simulink model "Robust_joint_Space"  (R2020b)
settings: Solver=VariableStepAuto  StartTime=0.0  StopTime=10  RelTol=1e-3
(part 4 of 7)

== matlab function Robust_joint_Space/plant/MATLAB Function4 ==
  data: M input; NumTerm input; Thetadd output
function Thetadd = Response(M,NumTerm)
Thetadd=M\NumTerm;

== matlab function Robust_joint_Space/plant/MATLAB Function2 ==
  data: Theta input; M output
function M = NumM(Theta)
t1=Theta(1);
t2=Theta(2);
t3=Theta(3);
t4=Theta(4);
t5=Theta(5);
t6=Theta(6);

L1=0.1025;
L2=0.408;
L3=0.376;
L4=0.1025; 
L5=0.1025;


M=zeros(6);
M(1)=(999498*cos(t3 + t4))/5 - (9799*L4)/40 - (33481296*cos(2*t2 + t3))/25 -...
    (30203396714246934648101547*cos(2*t2))/28823037615171174400 - (401759*cos(2*t2 + 2*t3 + 2*t4))/16 -...
    (15427656*cos(2*t2 + 2*t3))/25 - (999498*cos(2*t2 + t3 + t4))/5 - (219461*L1)/100 + (33481296*cos(t3))/25 +...
    (921106*cos(t4))/5 - (921106*cos(2*t2 + 2*t3 + t4))/5 - (239*L3^2*cos(2*t2 + 2*t3 + 2*t4 - 2*t5))/3200 -...
    (239*L3^2*cos(2*t2 + 2*t3 + 2*t4 + 2*t5))/3200 + (24378*L4*cos(2*t2 + t3 + t4))/25 +...
    (12189*L3*cos(t3 + t4 - t5))/50 - (757*L2^2*cos(2*t2))/800 + (239*L3^2*cos(2*t5))/1600 +...
    (239*L3^2*cos(2*t2 + 2*t3 + 2*t4))/1600 - (239*L4^2*cos(2*t2 + 2*t3 + 2*t4))/200 - (24378*L4*cos(t3 + t4))/25 -...
    (11233*L3*cos(t4 + t5))/50 - (11233*L3*cos(2*t2 + 2*t3 + t4 - t5))/50 + (9799*L3*cos(2*t2 + 2*t3 + 2*t4 + t5))/160 +...
    (67159*L3*cos(t5))/200 - (22466*L4*cos(t4))/25 + (22466*L4*cos(2*t2 + 2*t3 + t4))/25 +...
    (12189*L3*cos(2*t2 + t3 + t4 + t5))/50 + (781*L1^2)/100 + (757*L2^2)/800 + (717*L3^2)/1600 +...
    (239*L4^2)/200 + (11233*L3*cos(t4 - t5))/50 - (9799*L3*cos(2*t2 + 2*t3 + 2*t4 - t5))/160 -...
    (12189*L3*cos(t3 + t4 + t5))/50 + (9799*L4*cos(2*t2 + 2*t3 + 2*t4))/40 -...
    (12189*L3*cos(2*t2 + t3 + t4 - t5))/50 + (11233*L3*cos(2*t2 + 2*t3 + t4 + t5))/50 +...
    (239*L3*L4*cos(2*t2 + 2*t3 + 2*t4 - t5))/400 - (239*L3*L4*cos(2*t2 + 2*t3 + 2*t4 + t5))/400 +...
    60184539611691967063155889/28823037615171174400;
M(7)=(61463515545781917*cos(t1 + 2*t2))/2305843009213693952 - (61463515545781917*cos(t1 - 2*t2))/2305843009213693952 -...
    (2753519*cos(t2 + t3 + t4))/40 - (11529711*cos(t2 + t3))/25 - (18042729*cos(t2))/25 - (757*L2^2*cos(t1 - 2*t2))/1600 +...
    (757*L2^2*cos(t1 + 2*t2))/1600 - (11233*L3*cos(t2 + t3 - t5))/50 + (4541*L3*cos(t2 + t3 + t4 + t5))/200 -...
    (212717*L2*cos(t1 + t2))/800 + (7426*L1*cos(t2 + t3))/5 - (12189*L3*cos(t2 + t5))/50 + (79662*L1*cos(t2))/25 -...
    (58077*L3*cos(t2 + t3 + t4 - t5))/400 - (212717*L2*cos(t1 - t2))/800 - (12189*L3*cos(t2 - t5))/50 -...
    (11233*L3*cos(t2 + t3 + t5))/50 + (67159*L4*cos(t2 + t3 + t4))/200 - (239*L3^2*cos(t2 + t3 + t4 - 2*t5))/1600 +...
    (239*L3^2*cos(t2 + t3 + t4 + 2*t5))/1600 + (239*L3*L4*cos(t2 + t3 + t4 + t5))/400 +...
    (239*L3*L4*cos(t2 + t3 + t4 - t5))/400;
M(13)=(1690603261718859*cos(t1 - 2*t2))/2305843009213693952 - (1690603261718859*cos(t1 + 2*t2))/2305843009213693952 -...
    (2753519*cos(t2 + t3 + t4))/40 - (11529711*cos(t2 + t3))/25 - (11233*L3*cos(t2 + t3 - t5))/50 +...
    (4541*L3*cos(t2 + t3 + t4 + t5))/200 + (7426*L1*cos(t2 + t3))/5 - (58077*L3*cos(t2 + t3 + t4 - t5))/400 -...
    (11233*L3*cos(t2 + t3 + t5))/50 + (67159*L4*cos(t2 + t3 + t4))/200 - (239*L3^2*cos(t2 + t3 + t4 - 2*t5))/1600 +...
    (239*L3^2*cos(t2 + t3 + t4 + 2*t5))/1600 + (239*L3*L4*cos(t2 + t3 + t4 + t5))/400 +...
    (239*L3*L4*cos(t2 + t3 + t4 - t5))/400;
M(19)=(1690603261718859*cos(t1 - 2*t2))/2305843009213693952 - (1690603261718859*cos(t1 + 2*t2))/2305843009213693952 -...
    (2753519*cos(t2 + t3 + t4))/40 + (4541*L3*cos(t2 + t3 + t4 + t5))/200 - (58077*L3*cos(t2 + t3 + t4 - t5))/400 +...
    (67159*L4*cos(t2 + t3 + t4))/200 - (239*L3^2*cos(t2 + t3 + t4 - 2*t5))/1600 + (239*L3^2*cos(t2 + t3 + t4 + 2*t5))/1600 +...
    (239*L3*L4*cos(t2 + t3 + t4 + t5))/400 + (239*L3*L4*cos(t2 + t3 + t4 - t5))/400;
M(25)=(1690603261718859*cos(t2 + t3 + t4))/1152921504606846976 - (1690603261718859*cos(t1 + t2 - t3 - t4))/4611686018427387904 +...
    (1690603261718859*cos(3*t2 - t1 + t3 + t4))/4611686018427387904 - (1690603261718859*cos(t3 - t2 + t4))/2305843009213693952 -...
    (1690603261718859*cos(3*t2 + t3 + t4))/2305843009213693952 - (1690603261718859*cos(t1 - t2 + t3 + t4))/4611686018427387904 +...
    (1690603261718859*cos(t1 + 3*t2 + t3 + t4))/4611686018427387904 - (11233*L3*cos(t2 + t3 - t5))/50 + (239*L3^2*cos(t2 + t3 + t4))/400 +...
    (58077*L3*cos(t2 + t3 + t4 + t5))/400 + (12189*L3*cos(t2 + t5))/50 + (4541*L3*cos(t2 + t3 + t4 - t5))/200 - (12189*L3*cos(t2 - t5))/50 +...
    (11233*L3*cos(t2 + t3 + t5))/50 - (239*L3*L4*cos(t2 + t3 + t4 + t5))/400 + (239*L3*L4*cos(t2 + t3 + t4 - t5))/400;
M(31)=0;
M(2)=(61463515545781917*cos(t1 + 2*t2))/2305843009213693952 - (61463515545781917*cos(t1 - 2*t2))/2305843009213693952 -...
    (2753519*cos(t2 + t3 + t4))/40 - (11529711*cos(t2 + t3))/25 - (18042729*cos(t2))/25 - (757*L2^2*cos(t1 - 2*t2))/1600 +...
    (757*L2^2*cos(t1 + 2*t2))/1600 - (11233*L3*cos(t2 + t3 - t5))/50 + (4541*L3*cos(t2 + t3 + t4 + t5))/200 -...
    (212717*L2*cos(t1 + t2))/800 + (7426*L1*cos(t2 + t3))/5 - (12189*L3*cos(t2 + t5))/50 + (79662*L1*cos(t2))/25 -...
    (58077*L3*cos(t2 + t3 + t4 - t5))/400 - (212717*L2*cos(t1 - t2))/800 - (12189*L3*cos(t2 - t5))/50 -...
    (11233*L3*cos(t2 + t3 + t5))/50 + (67159*L4*cos(t2 + t3 + t4))/200 - (239*L3^2*cos(t2 + t3 + t4 - 2*t5))/1600 +...
    (239*L3^2*cos(t2 + t3 + t4 + 2*t5))/1600 + (239*L3*L4*cos(t2 + t3 + t4 + t5))/400 + (239*L3*L4*cos(t2 + t3 + t4 - t5))/400;
M(8)=(66962592*cos(t3))/25 - (9799*L4)/20 + (1842212*cos(t4))/5 + (1998996*cos(t3)*cos(t4))/5 - (1998996*sin(t3)*sin(t4))/5 -...
    (17228543827841635967893663*cos(t1)^2)/115292150460684697600 - (61463515545781917*cos(t2)^2)/576460752303423488 +...
    (1690603261718859*cos(t3)^2)/576460752303423488 + (757*L2^2*cos(t1)^2)/400 + (757*L2^2*cos(t2)^2)/400 -...
    (239*L3^2*cos(t5)^2)/400 - (44932*L4*cos(t4))/25 + (239*L3^2)/400 + (239*L4^2)/100 + ...
    (61463515545781917*cos(t1)^2*cos(t2)^2)/576460752303423488 - (1690603261718859*cos(t1)^2*cos(t3)^2)/288230376151711744 -...
    (48756*L4*cos(t3)*cos(t4))/25 - (757*L2^2*cos(t1)^2*cos(t2)^2)/400 + (48756*L4*sin(t3)*sin(t4))/25 + (22466*L3*sin(t4)*sin(t5))/25 -...
    (212717*L2*cos(t1)*sin(t1)*sin(t2))/200 + (24378*L3*cos(t3)*sin(t4)*sin(t5))/25 + (24378*L3*cos(t4)*sin(t3)*sin(t5))/25 -...
    (1690603261718859*cos(t1)*cos(t3)*sin(t1)*sin(t3))/288230376151711744 + 406940712223380376880235337/115292150460684697600;
M(14)=(33481296*cos(t3))/25 - (9799*L4)/20 + (1842212*cos(t4))/5 + (999498*cos(t3)*cos(t4))/5 - (999498*sin(t3)*sin(t4))/5 +...
    (22503512638915017*cos(t1)^2)/4611686018427387904 + (1690603261718859*cos(t2)^2)/576460752303423488 +...
    (1690603261718859*cos(t3)^2)/576460752303423488 - (239*L3^2*cos(t5)^2)/400 - (44932*L4*cos(t4))/25 +...
    (239*L3^2)/400 + (239*L4^2)/100 - (1690603261718859*cos(t1)^2*cos(t2)^2)/576460752303423488 -...
    (1690603261718859*cos(t1)^2*cos(t3)^2)/288230376151711744 - (24378*L4*cos(t3)*cos(t4))/25 +...
    (24378*L4*sin(t3)*sin(t4))/25 + (22466*L3*sin(t4)*sin(t5))/25 + (12189*L3*cos(t3)*sin(t4)*sin(t5))/25 +...
    (12189*L3*cos(t4)*sin(t3)*sin(t5))/25 - (1690603261718859*cos(t1)*cos(t3)*sin(t1)*sin(t3))/288230376151711744 +...
    148084969195448577098115273/115292150460684697600;
M(20)=(24162136260015883*cos(2*t1))/9223372036854775808 - (9799*L4)/20 + (1690603261718859*cos(2*t2))/2305843009213693952 +...
    (921106*cos(t4))/5 + (999498*cos(t3)*cos(t4))/5 - (999498*sin(t3)*sin(t4))/5 - (239*L3^2*cos(t5)^2)/400 -...
    (22466*L4*cos(t4))/25 + (239*L3^2)/400 + (239*L4^2)/100 - (1690603261718859*cos(2*t1)*cos(2*t2))/2305843009213693952 -...
    (1690603261718859*cos(2*t1)*cos(t3)^2)/576460752303423488 - (24378*L4*cos(t3)*cos(t4))/25 -...
    (1690603261718859*sin(2*t1)*cos(t3)*sin(t3))/576460752303423488 + (24378*L4*sin(t3)*sin(t4))/25 +...
    (11233*L3*sin(t4)*sin(t5))/25 + (12189*L3*cos(t3)*sin(t4)*sin(t5))/25 + (12189*L3*cos(t4)*sin(t3)*sin(t5))/25 +...
    463196680911590935827689/9223372036854775808;
M(26)=(1690603261718859*cos(2*t1 + t2 - t3 + t4))/2305843009213693952 - (1690603261718859*cos(t1 + t2 - t3 - t4))/4611686018427387904 +...
    (1690603261718859*cos(2*t1 - t2 + t3 + t4))/9223372036854775808 + (1690603261718859*cos(3*t2 - t1 + t3 + t4))/4611686018427387904 -...
    (1690603261718859*cos(t2 - 2*t1 + 3*t3 + t4))/2305843009213693952 - (1690603261718859*cos(3*t2 - 2*t1 + t3 + t4))/9223372036854775808 +...
    (1690603261718859*cos(2*t1 + 3*t2 + t3 + t4))/9223372036854775808 - (1690603261718859*cos(2*t1 + t2 - t3 - t4))/9223372036854775808 +...
    (1690603261718859*cos(t1 - t2 + t3 + t4))/4611686018427387904 + (10637310166265011*cos(t2 - 2*t1 + t3 + t4))/18446744073709551616 -...
    (10637310166265011*cos(2*t1 + t2 + t3 + t4))/18446744073709551616 - (1690603261718859*cos(t1 + 3*t2 + t3 + t4))/4611686018427387904 -...
    (12189*L3*cos(t3 + t4 - t5))/50 - (11233*L3*cos(t4 + t5))/50 - (9799*L3*cos(t5))/80 - (11233*L3*cos(t4 - t5))/50 -...
    (12189*L3*cos(t3 + t4 + t5))/50 + (239*L3*L4*cos(t5))/200;
M(32)=(3874897119389575*cos(t5))/4611686018427387904 + (3874897119389575*cos(t1)^2*cos(t5))/4611686018427387904 -...
    (3874897119389575*cos(t1)*cos(t2)*cos(t3)*cos(t4)*sin(t1)*sin(t5))/4611686018427387904 +...
    (3874897119389575*cos(t1)*cos(t2)*sin(t1)*sin(t3)*sin(t4)*sin(t5))/4611686018427387904 +...
    (3874897119389575*cos(t1)*cos(t3)*sin(t1)*sin(t2)*sin(t4)*sin(t5))/4611686018427387904 +...
    (3874897119389575*cos(t1)*cos(t4)*sin(t1)*sin(t2)*sin(t3)*sin(t5))/4611686018427387904;
M(3)=(1690603261718859*cos(t1 - 2*t2))/2305843009213693952 - (1690603261718859*cos(t1 + 2*t2))/2305843009213693952 -...
    (2753519*cos(t2 + t3 + t4))/40 - (11529711*cos(t2 + t3))/25 - (11233*L3*cos(t2 + t3 - t5))/50 +...
    (4541*L3*cos(t2 + t3 + t4 + t5))/200 + (7426*L1*cos(t2 + t3))/5 - (58077*L3*cos(t2 + t3 + t4 - t5))/400 -...
    (11233*L3*cos(t2 + t3 + t5))/50 + (67159*L4*cos(t2 + t3 + t4))/200 - (239*L3^2*cos(t2 + t3 + t4 - 2*t5))/1600 +...
    (239*L3^2*cos(t2 + t3 + t4 + 2*t5))/1600 + (239*L3*L4*cos(t2 + t3 + t4 + t5))/400 +...
    (239*L3*L4*cos(t2 + t3 + t4 - t5))/400;
M(9)=(33481296*cos(t3))/25 - (9799*L4)/20 + (1842212*cos(t4))/5 + (999498*cos(t3)*cos(t4))/5 - (999498*sin(t3)*sin(t4))/5 +...
    (22503512638915017*cos(t1)^2)/4611686018427387904 + (1690603261718859*cos(t2)^2)/576460752303423488 + ...
    (1690603261718859*cos(t3)^2)/576460752303423488 - (239*L3^2*cos(t5)^2)/400 - (44932*L4*cos(t4))/25 + ...
    (239*L3^2)/400 + (239*L4^2)/100 - (1690603261718859*cos(t1)^2*cos(t2)^2)/576460752303423488 - ...
    (1690603261718859*cos(t1)^2*cos(t3)^2)/288230376151711744 - (24378*L4*cos(t3)*cos(t4))/25 + ...
    (24378*L4*sin(t3)*sin(t4))/25 + (22466*L3*sin(t4)*sin(t5))/25 + (12189*L3*cos(t3)*sin(t4)*sin(t5))/25 +...
    (12189*L3*cos(t4)*sin(t3)*sin(t5))/25 - (1690603261718859*cos(t1)*cos(t3)*sin(t1)*sin(t3))/288230376151711744 +...
    148084969195448577098115273/115292150460684697600;
M(15)=(1842212*cos(t4))/5 - (9799*L4)/20 + (22503512638915017*cos(t1)^2)/4611686018427387904 +...
    (1690603261718859*cos(t2)^2)/576460752303423488 + (1690603261718859*cos(t3)^2)/576460752303423488 -...
    (239*L3^2*cos(t5)^2)/400 - (44932*L4*cos(t4))/25 + (239*L3^2)/400 + (239*L4^2)/100 -...
    (1690603261718859*cos(t1)^2*cos(t2)^2)/576460752303423488 - (1690603261718859*cos(t1)^2*cos(t3)^2)/288230376151711744 +...
    (22466*L3*sin(t4)*sin(t5))/25 - (1690603261718859*cos(t1)*cos(t3)*sin(t1)*sin(t3))/288230376151711744 +...
    148084969195448577098115273/115292150460684697600;
M(21)=(921106*cos(t4))/5 - (9799*L4)/20 + (30924549306891319*cos(t1)^2)/4611686018427387904 +...
    (1690603261718859*cos(t2)^2)/576460752303423488 + (1690603261718859*cos(t3)^2)/576460752303423488 -...
    (239*L3^2*cos(t5)^2)/400 - (22466*L4*cos(t4))/25 + (239*L3^2)/400 + (239*L4^2)/100 -...
    (1690603261718859*cos(t1)^2*cos(t2)^2)/576460752303423488 - (1690603261718859*cos(t1)^2*cos(t3)^2)/288230376151711744 +...
    (11233*L3*sin(t4)*sin(t5))/25 - (1690603261718859*cos(t1)*cos(t3)*sin(t1)*sin(t3))/288230376151711744 + 231598321612314291030467/4611686018427387904;
M(27)=(1690603261718859*cos(2*t1 + t2 - t3 + t4))/2305843009213693952 - (1690603261718859*cos(t1 + t2 - t3 - t4))/4611686018427387904 +...
    (1690603261718859*cos(2*t1 - t2 + t3 + t4))/9223372036854775808 + (1690603261718859*cos(3*t2 - t1 + t3 + t4))/4611686018427387904 -...
    (1690603261718859*cos(t2 - 2*t1 + 3*t3 + t4))/2305843009213693952 - (1690603261718859*cos(3*t2 - 2*t1 + t3 + t4))/9223372036854775808 +...
    (1690603261718859*cos(2*t1 + 3*t2 + t3 + t4))/9223372036854775808 - (1690603261718859*cos(2*t1 + t2 - t3 - t4))/9223372036854775808 +...
    (1690603261718859*cos(t1 - t2 + t3 + t4))/4611686018427387904 + (10637310166265011*cos(t2 - 2*t1 + t3 + t4))/18446744073709551616 -...
    (10637310166265011*cos(2*t1 + t2 + t3 + t4))/18446744073709551616 - (1690603261718859*cos(t1 + 3*t2 + t3 + t4))/4611686018427387904 -...
    (11233*L3*cos(t4 + t5))/50 - (9799*L3*cos(t5))/80 - (11233*L3*cos(t4 - t5))/50 + (239*L3*L4*cos(t5))/200;
M(33)=(3874897119389575*cos(t5))/4611686018427387904 + (3874897119389575*cos(t1)^2*cos(t5))/4611686018427387904 -...
    (3874897119389575*cos(t1)*cos(t2)*cos(t3)*cos(t4)*sin(t1)*sin(t5))/4611686018427387904 +...
    (3874897119389575*cos(t1)*cos(t2)*sin(t1)*sin(t3)*sin(t4)*sin(t5))/4611686018427387904 +...
    (3874897119389575*cos(t1)*cos(t3)*sin(t1)*sin(t2)*sin(t4)*sin(t5))/4611686018427387904 +...
    (3874897119389575*cos(t1)*cos(t4)*sin(t1)*sin(t2)*sin(t3)*sin(t5))/4611686018427387904;
M(4)=(1690603261718859*cos(t1 - 2*t2))/2305843009213693952 - (1690603261718859*cos(t1 + 2*t2))/2305843009213693952 -...
    (2753519*cos(t2 + t3 + t4))/40 + (4541*L3*cos(t2 + t3 + t4 + t5))/200 - (58077*L3*cos(t2 + t3 + t4 - t5))/400 +...
    (67159*L4*cos(t2 + t3 + t4))/200 - (239*L3^2*cos(t2 + t3 + t4 - 2*t5))/1600 + (239*L3^2*cos(t2 + t3 + t4 + 2*t5))/1600 +...
    (239*L3*L4*cos(t2 + t3 + t4 + t5))/400 + (239*L3*L4*cos(t2 + t3 + t4 - t5))/400;
M(10)=(24162136260015883*cos(2*t1))/9223372036854775808 - (9799*L4)/20 + (1690603261718859*cos(2*t2))/2305843009213693952 +...
    (921106*cos(t4))/5 + (999498*cos(t3)*cos(t4))/5 - (999498*sin(t3)*sin(t4))/5 - (239*L3^2*cos(t5)^2)/400 - (22466*L4*cos(t4))/25 +...
    (239*L3^2)/400 + (239*L4^2)/100 - (1690603261718859*cos(2*t1)*cos(2*t2))/2305843009213693952 -...
    (1690603261718859*cos(2*t1)*cos(t3)^2)/576460752303423488 - (24378*L4*cos(t3)*cos(t4))/25 -...
    (1690603261718859*sin(2*t1)*cos(t3)*sin(t3))/576460752303423488 + (24378*L4*sin(t3)*sin(t4))/25 + (11233*L3*sin(t4)*sin(t5))/25 +...
    (12189*L3*cos(t3)*sin(t4)*sin(t5))/25 + (12189*L3*cos(t4)*sin(t3)*sin(t5))/25 + 463196680911590935827689/9223372036854775808;
M(16)=(921106*cos(t4))/5 - (9799*L4)/20 + (30924549306891319*cos(t1)^2)/4611686018427387904 +...
    (1690603261718859*cos(t2)^2)/576460752303423488 + (1690603261718859*cos(t3)^2)/576460752303423488 -...
    (239*L3^2*cos(t5)^2)/400 - (22466*L4*cos(t4))/25 + (239*L3^2)/400 + (239*L4^2)/100 -...
    (1690603261718859*cos(t1)^2*cos(t2)^2)/576460752303423488 - (1690603261718859*cos(t1)^2*cos(t3)^2)/288230376151711744 +...
    (11233*L3*sin(t4)*sin(t5))/25 - (1690603261718859*cos(t1)*cos(t3)*sin(t1)*sin(t3))/288230376151711744 +...
    231598321612314291030467/4611686018427387904;
M(22)=(10637310166265011*cos(2*t1))/9223372036854775808 - (9799*L4)/20 + (1690603261718859*cos(2*t2))/2305843009213693952 -...
    (239*L3^2*cos(2*t5))/800 + (239*L3^2)/800 + (239*L4^2)/100 - (1690603261718859*cos(2*t1)*cos(2*t2))/2305843009213693952 -...
    (1690603261718859*cos(2*t1)*cos(2*t3))/1152921504606846976 - (1690603261718859*sin(2*t1)*sin(2*t3))/1152921504606846976 +...
    463196680911590935827689/9223372036854775808;
M(28)=(1690603261718859*cos(2*t1 + t2 - t3 + t4))/2305843009213693952 - (1690603261718859*cos(t1 + t2 - t3 - t4))/4611686018427387904 +...
    (1690603261718859*cos(2*t1 - t2 + t3 + t4))/9223372036854775808 + (1690603261718859*cos(3*t2 - t1 + t3 + t4))/4611686018427387904 -...
    (1690603261718859*cos(t2 - 2*t1 + 3*t3 + t4))/2305843009213693952 - (1690603261718859*cos(3*t2 - 2*t1 + t3 + t4))/9223372036854775808 +...
    (1690603261718859*cos(2*t1 + 3*t2 + t3 + t4))/9223372036854775808 - (1690603261718859*cos(2*t1 + t2 - t3 - t4))/9223372036854775808 +...
    (1690603261718859*cos(t1 - t2 + t3 + t4))/4611686018427387904 + (10637310166265011*cos(t2 - 2*t1 + t3 + t4))/18446744073709551616 -...
    (10637310166265011*cos(2*t1 + t2 + t3 + t4))/18446744073709551616 - (1690603261718859*cos(t1 + 3*t2 + t3 + t4))/4611686018427387904 -...
    (9799*L3*cos(t5))/80 + (239*L3*L4*cos(t5))/200;
M(34)=(3874897119389575*cos(t5))/4611686018427387904 + (3874897119389575*cos(t1)^2*cos(t5))/4611686018427387904 -...
    (3874897119389575*cos(t1)*cos(t2)*cos(t3)*cos(t4)*sin(t1)*sin(t5))/4611686018427387904 +...
    (3874897119389575*cos(t1)*cos(t2)*sin(t1)*sin(t3)*sin(t4)*sin(t5))/4611686018427387904 +...
    (3874897119389575*cos(t1)*cos(t3)*sin(t1)*sin(t2)*sin(t4)*sin(t5))/4611686018427387904 +...
    (3874897119389575*cos(t1)*cos(t4)*sin(t1)*sin(t2)*sin(t3)*sin(t5))/4611686018427387904;
M(5)=(1690603261718859*cos(t2 + t3 + t4))/1152921504606846976 -...
    (1690603261718859*cos(t1 + t2 - t3 - t4))/4611686018427387904 +...
    (1690603261718859*cos(3*t2 - t1 + t3 + t4))/4611686018427387904 -...
    (1690603261718859*cos(t3 - t2 + t4))/2305843009213693952 - (1690603261718859*cos(3*t2 + t3 + t4))/2305843009213693952 -...
    (1690603261718859*cos(t1 - t2 + t3 + t4))/4611686018427387904 +...
    (1690603261718859*cos(t1 + 3*t2 + t3 + t4))/4611686018427387904 - (11233*L3*cos(t2 + t3 - t5))/50 +...
    (239*L3^2*cos(t2 + t3 + t4))/400 + (58077*L3*cos(t2 + t3 + t4 + t5))/400 + (12189*L3*cos(t2 + t5))/50 +...
    (4541*L3*cos(t2 + t3 + t4 - t5))/200 - (12189*L3*cos(t2 - t5))/50 + (11233*L3*cos(t2 + t3 + t5))/50 -...
    (239*L3*L4*cos(t2 + t3 + t4 + t5))/400 + (239*L3*L4*cos(t2 + t3 + t4 - t5))/400;
M(11)=(1690603261718859*cos(2*t1 + t2 - t3 + t4))/2305843009213693952 - (1690603261718859*cos(t1 + t2 - t3 - t4))/4611686018427387904 +...
    (1690603261718859*cos(2*t1 - t2 + t3 + t4))/9223372036854775808 + (1690603261718859*cos(3*t2 - t1 + t3 + t4))/4611686018427387904 -...
    (1690603261718859*cos(t2 - 2*t1 + 3*t3 + t4))/2305843009213693952 - (1690603261718859*cos(3*t2 - 2*t1 + t3 + t4))/9223372036854775808 +...
    (1690603261718859*cos(2*t1 + 3*t2 + t3 + t4))/9223372036854775808 - (1690603261718859*cos(2*t1 + t2 - t3 - t4))/9223372036854775808 +...
    (1690603261718859*cos(t1 - t2 + t3 + t4))/4611686018427387904 + (10637310166265011*cos(t2 - 2*t1 + t3 + t4))/18446744073709551616 -...
    (10637310166265011*cos(2*t1 + t2 + t3 + t4))/18446744073709551616 - (1690603261718859*cos(t1 + 3*t2 + t3 + t4))/4611686018427387904 -...
    (12189*L3*cos(t3 + t4 - t5))/50 - (11233*L3*cos(t4 + t5))/50 - (9799*L3*cos(t5))/80 - (11233*L3*cos(t4 - t5))/50 -...
    (12189*L3*cos(t3 + t4 + t5))/50 + (239*L3*L4*cos(t5))/200;
M(17)=(1690603261718859*cos(2*t1 + t2 - t3 + t4))/2305843009213693952 - (1690603261718859*cos(t1 + t2 - t3 - t4))/4611686018427387904 +...
    (1690603261718859*cos(2*t1 - t2 + t3 + t4))/9223372036854775808 + (1690603261718859*cos(3*t2 - t1 + t3 + t4))/4611686018427387904 -...
    (1690603261718859*cos(t2 - 2*t1 + 3*t3 + t4))/2305843009213693952 - (1690603261718859*cos(3*t2 - 2*t1 + t3 + t4))/9223372036854775808 +...
    (1690603261718859*cos(2*t1 + 3*t2 + t3 + t4))/9223372036854775808 - (1690603261718859*cos(2*t1 + t2 - t3 - t4))/9223372036854775808 +...
    (1690603261718859*cos(t1 - t2 + t3 + t4))/4611686018427387904 + (10637310166265011*cos(t2 - 2*t1 + t3 + t4))/18446744073709551616 -...
    (10637310166265011*cos(2*t1 + t2 + t3 + t4))/18446744073709551616 - (1690603261718859*cos(t1 + 3*t2 + t3 + t4))/4611686018427387904 -...
    (11233*L3*cos(t4 + t5))/50 - (9799*L3*cos(t5))/80 - (11233*L3*cos(t4 - t5))/50 + (239*L3*L4*cos(t5))/200;
M(23)=(1690603261718859*cos(2*t1 + t2 - t3 + t4))/2305843009213693952 - (1690603261718859*cos(t1 + t2 - t3 - t4))/4611686018427387904 +...
    (1690603261718859*cos(2*t1 - t2 + t3 + t4))/9223372036854775808 + (1690603261718859*cos(3*t2 - t1 + t3 + t4))/4611686018427387904 -...
    (1690603261718859*cos(t2 - 2*t1 + 3*t3 + t4))/2305843009213693952 - (1690603261718859*cos(3*t2 - 2*t1 + t3 + t4))/9223372036854775808 +...
    (1690603261718859*cos(2*t1 + 3*t2 + t3 + t4))/9223372036854775808 - (1690603261718859*cos(2*t1 + t2 - t3 - t4))/9223372036854775808 +...
    (1690603261718859*cos(t1 - t2 + t3 + t4))/4611686018427387904 + (10637310166265011*cos(t2 - 2*t1 + t3 + t4))/18446744073709551616 -...
    (10637310166265011*cos(2*t1 + t2 + t3 + t4))/18446744073709551616 - (1690603261718859*cos(t1 + 3*t2 + t3 + t4))/4611686018427387904 -...
    (9799*L3*cos(t5))/80 + (239*L3*L4*cos(t5))/200;
M(29)=(239*L3^2)/400 + (10637310166265011*cos(2*t2 - 2*t1 + 2*t3 + 2*t4))/36893488147419103232 +...
    (10637310166265011*cos(2*t1 + 2*t2 + 2*t3 + 2*t4))/36893488147419103232 + (1690603261718859*cos(4*t2 - t1 + 2*t3 + 2*t4))/4611686018427387904 -...
    (1690603261718859*cos(2*t2 - 2*t1 + 4*t3 + 2*t4))/4611686018427387904 - (1690603261718859*cos(4*t2 - 2*t1 + 2*t3 + 2*t4))/18446744073709551616 -...
    (1690603261718859*cos(2*t1 + 4*t2 + 2*t3 + 2*t4))/18446744073709551616 - (10637310166265011*cos(2*t1))/18446744073709551616 -...
    (1690603261718859*cos(2*t2))/4611686018427387904 - (1690603261718859*cos(2*t3 - t1 + 2*t4))/4611686018427387904 -...
    (1690603261718859*cos(2*t1 + 2*t2 + 2*t4))/4611686018427387904 - (1690603261718859*cos(2*t3 - 2*t1 + 2*t4))/18446744073709551616 -...
    (1690603261718859*cos(2*t1 + 2*t3 + 2*t4))/18446744073709551616 - (31911930498795033*cos(2*t2 + 2*t3 + 2*t4))/18446744073709551616 -...
    (5071809785156577*cos(4*t2 + 2*t3 + 2*t4))/9223372036854775808 + (1690603261718859*cos(2*t1 - 2*t2))/9223372036854775808 +...
    (1690603261718859*cos(2*t1 + 2*t2))/9223372036854775808 + (1690603261718859*cos(2*t1 - 2*t3))/2305843009213693952 -...
    (5071809785156577*cos(2*t3 + 2*t4))/9223372036854775808 + (1690603261718859*cos(t1 + 4*t2 + 2*t3 + 2*t4))/4611686018427387904 -...
    (1690603261718859*cos(t1 + 2*t3 + 2*t4))/4611686018427387904 + 58961582686296777/18446744073709551616;
M(35)=(11624691358168725*sin(2*t2)*sin(2*t3)*sin(2*t4)*sin(t5))/18446744073709551616 - (11624691358168725*cos(2*t2)*cos(2*t3)*sin(2*t4)*sin(t5))/18446744073709551616 -...
    (11624691358168725*cos(2*t2)*cos(2*t4)*sin(2*t3)*sin(t5))/18446744073709551616 - (11624691358168725*cos(2*t3)*cos(2*t4)*sin(2*t2)*sin(t5))/18446744073709551616 +...
    (3874897119389575*sin(2*t1)*cos(t2)*cos(t3)*cos(t5)*sin(t4))/9223372036854775808 + (3874897119389575*sin(2*t1)*cos(t2)*cos(t4)*cos(t5)*sin(t3))/9223372036854775808 +...
    (3874897119389575*sin(2*t1)*cos(t3)*cos(t4)*cos(t5)*sin(t2))/9223372036854775808 + (3874897119389575*cos(2*t1)*cos(2*t2)*cos(2*t3)*sin(2*t4)*sin(t5))/18446744073709551616 +...
    (3874897119389575*cos(2*t1)*cos(2*t2)*cos(2*t4)*sin(2*t3)*sin(t5))/18446744073709551616 + (3874897119389575*cos(2*t1)*cos(2*t3)*cos(2*t4)*sin(2*t2)*sin(t5))/18446744073709551616 -...
    (3874897119389575*sin(2*t1)*cos(t5)*sin(t2)*sin(t3)*sin(t4))/9223372036854775808 - (3874897119389575*cos(2*t1)*sin(2*t2)*sin(2*t3)*sin(2*t4)*sin(t5))/18446744073709551616;
M(6)=0;
M(12)=(3874897119389575*cos(t5))/4611686018427387904 + (3874897119389575*cos(t1)^2*cos(t5))/4611686018427387904 -...
    (3874897119389575*cos(t1)*cos(t2)*cos(t3)*cos(t4)*sin(t1)*sin(t5))/4611686018427387904 + (3874897119389575*cos(t1)*cos(t2)*sin(t1)*sin(t3)*sin(t4)*sin(t5))/4611686018427387904 +...
    (3874897119389575*cos(t1)*cos(t3)*sin(t1)*sin(t2)*sin(t4)*sin(t5))/4611686018427387904 + (3874897119389575*cos(t1)*cos(t4)*sin(t1)*sin(t2)*sin(t3)*sin(t5))/4611686018427387904;
M(18)=(3874897119389575*cos(t5))/4611686018427387904 + (3874897119389575*cos(t1)^2*cos(t5))/4611686018427387904 - (3874897119389575*cos(t1)*cos(t2)*cos(t3)*cos(t4)*sin(t1)*sin(t5))/4611686018427387904 +...
    (3874897119389575*cos(t1)*cos(t2)*sin(t1)*sin(t3)*sin(t4)*sin(t5))/4611686018427387904 + (3874897119389575*cos(t1)*cos(t3)*sin(t1)*sin(t2)*sin(t4)*sin(t5))/4611686018427387904 +...
    (3874897119389575*cos(t1)*cos(t4)*sin(t1)*sin(t2)*sin(t3)*sin(t5))/4611686018427387904;
M(24)=(3874897119389575*cos(t5))/4611686018427387904 + (3874897119389575*cos(t1)^2*cos(t5))/4611686018427387904 - (3874897119389575*cos(t1)*cos(t2)*cos(t3)*cos(t4)*sin(t1)*sin(t5))/4611686018427387904 +...
    (3874897119389575*cos(t1)*cos(t2)*sin(t1)*sin(t3)*sin(t4)*sin(t5))/4611686018427387904 + (3874897119389575*cos(t1)*cos(t3)*sin(t1)*sin(t2)*sin(t4)*sin(t5))/4611686018427387904 +...
    (3874897119389575*cos(t1)*cos(t4)*sin(t1)*sin(t2)*sin(t3)*sin(t5))/4611686018427387904;
M(30)=(11624691358168725*sin(2*t2)*sin(2*t3)*sin(2*t4)*sin(t5))/18446744073709551616 - (11624691358168725*cos(2*t2)*cos(2*t3)*sin(2*t4)*sin(t5))/18446744073709551616 -...
    (11624691358168725*cos(2*t2)*cos(2*t4)*sin(2*t3)*sin(t5))/18446744073709551616 - (11624691358168725*cos(2*t3)*cos(2*t4)*sin(2*t2)*sin(t5))/18446744073709551616 +...
    (3874897119389575*sin(2*t1)*cos(t2)*cos(t3)*cos(t5)*sin(t4))/9223372036854775808 + (3874897119389575*sin(2*t1)*cos(t2)*cos(t4)*cos(t5)*sin(t3))/9223372036854775808 +...
    (3874897119389575*sin(2*t1)*cos(t3)*cos(t4)*cos(t5)*sin(t2))/9223372036854775808 + (3874897119389575*cos(2*t1)*cos(2*t2)*cos(2*t3)*sin(2*t4)*sin(t5))/18446744073709551616 +...
    (3874897119389575*cos(2*t1)*cos(2*t2)*cos(2*t4)*sin(2*t3)*sin(t5))/18446744073709551616 + (3874897119389575*cos(2*t1)*cos(2*t3)*cos(2*t4)*sin(2*t2)*sin(t5))/18446744073709551616 -...
    (3874897119389575*sin(2*t1)*cos(t5)*sin(t2)*sin(t3)*sin(t4))/9223372036854775808 - (3874897119389575*cos(2*t1)*sin(2*t2)*sin(2*t3)*sin(2*t4)*sin(t5))/18446744073709551616;
M(36)=((3874897119389575*cos(t1)*cos(t2)*sin(t3)*sin(t4)*sin(t5))/4611686018427387904 - (3874897119389575*cos(t1)*cos(t2)*cos(t3)*cos(t4)*sin(t5))/4611686018427387904 -...
    (3874897119389575*cos(t5)*sin(t1))/4611686018427387904 + (3874897119389575*cos(t1)*cos(t3)*sin(t2)*sin(t4)*sin(t5))/4611686018427387904 +...
    (3874897119389575*cos(t1)*cos(t4)*sin(t2)*sin(t3)*sin(t5))/4611686018427387904)*(cos(t1)*cos(t2)*sin(t3)*sin(t4)*sin(t5) - cos(t1)*cos(t2)*cos(t3)*cos(t4)*sin(t5) -...
    cos(t5)*sin(t1) + cos(t1)*cos(t3)*sin(t2)*sin(t4)*sin(t5) + cos(t1)*cos(t4)*sin(t2)*sin(t3)*sin(t5)) + ((3874897119389575*cos(t1)*cos(t5))/2305843009213693952 -...
    (3874897119389575*cos(t2)*cos(t3)*cos(t4)*sin(t1)*sin(t5))/2305843009213693952 + (3874897119389575*cos(t2)*sin(t1)*sin(t3)*sin(t4)*sin(t5))/2305843009213693952 +...
    (3874897119389575*cos(t3)*sin(t1)*sin(t2)*sin(t4)*sin(t5))/2305843009213693952 + (3874897119389575*cos(t4)*sin(t1)*sin(t2)*sin(t3)*sin(t5))/2305843009213693952)*(cos(t1)*cos(t5) -...
    cos(t2)*cos(t3)*cos(t4)*sin(t1)*sin(t5) + cos(t2)*sin(t1)*sin(t3)*sin(t4)*sin(t5) + cos(t3)*sin(t1)*sin(t2)*sin(t4)*sin(t5) + cos(t4)*sin(t1)*sin(t2)*sin(t3)*sin(t5));

== matlab function Robust_joint_Space/plant/MATLAB Function ==
  data: Theta input; G output
function G = NumG(Theta)
t1=Theta(1);
t2=Theta(2);
t3=Theta(3);
t4=Theta(4);
t5=Theta(5);
t6=Theta(6);

L1=0.1025;
L2=0.408;
L3=0.376;
L4=0.1025; 
L5=0.1025;

G=[0
   5.8614750000000004348521542851813*L3*sin(t2 + t3 + t4 + t5) - 32201.128800000001308035280089825*sin(t2 + t3) - 50391.223200000000709678715793416*sin(t2) - 4806.4095000000003565787665138487*sin(t2 + t3 + t4) - 37.130850000000002353317540837452*L2*sin(t2) - 5.8614750000000004348521542851813*L3*sin(t2 + t3 + t4 - t5) + 23.445900000000001739408617140725*L4*sin(t2 + t3 + t4)
   5.8614750000000004348521542851813*L3*sin(t2 + t3 + t4 + t5) - 32201.128800000001308035280089825*sin(t2 + t3) - 4806.4095000000003565787665138487*sin(t2 + t3 + t4) - 5.8614750000000004348521542851813*L3*sin(t2 + t3 + t4 - t5) + 23.445900000000001739408617140725*L4*sin(t2 + t3 + t4)
   5.8614750000000004348521542851813*L3*sin(t2 + t3 + t4 + t5) - 4806.4095000000003565787665138487*sin(t2 + t3 + t4) - 5.8614750000000004348521542851813*L3*sin(t2 + t3 + t4 - t5) + 23.445900000000001739408617140725*L4*sin(t2 + t3 + t4)
   5.8614750000000004348521542851813*L3*sin(t2 + t3 + t4 + t5) + 5.8614750000000004348521542851813*L3*sin(t2 + t3 + t4 - t5)
   0];

== matlab function Robust_joint_Space/robust inverse dynamic controller/g_hat_prod ==
  data: m input; theta input; Ghat output
function Ghat = Find_G(m,theta)

m1 = m(1);
m2 = m(2);
m3 = m(3);
m4 = m(4);
m5 = m(5);
m6 = m(6);

t1 = theta(1);
t2 = theta(2);
t3 = theta(3);
t4 = theta(4);
t5 = theta(5);
t6 = theta(6);

L1=0.1025;
L2=0.408;
L3=0.376;
L4=0.1025; 
L5=0.1025;

Ghat = [0; 9.81*L4*m5*sin(t2 + t3 + t4) - 3688.56*m5*sin(t2 + t3) - 3688.56*m6*sin(t2 + t3) - 4002.48*m3*sin(t2) - 4002.48*m4*sin(t2) - 4002.48*m5*sin(t2) - 4002.48*m6*sin(t2) - 1005.525*m5*sin(t2 + t3 + t4) - 1005.525*m6*sin(t2 + t3 + t4) - 2.4525*L3*m5*sin(t2 + t3 + t4 - t5) - 3688.56*m4*sin(t2 + t3) + 2.4525*L3*m5*sin(t2 + t3 + t4 + t5) - 4.905*L2*m2*sin(t2); 9.81*L4*m5*sin(t2 + t3 + t4) - 3688.56*m5*sin(t2 + t3) - 3688.56*m6*sin(t2 + t3) - 1005.525*m5*sin(t2 + t3 + t4) - 1005.525*m6*sin(t2 + t3 + t4) - 2.4525*L3*m5*sin(t2 + t3 + t4 - t5) - 3688.56*m4*sin(t2 + t3) + 2.4525*L3*m5*sin(t2 + t3 + t4 + t5); - 9.81*m5*(102.5*sin(t2 + t3 + t4) - 0.25*L3*sin(t2 + t3 + t4 + t5) - 1.0*L4*sin(t2 + t3 + t4) + 0.25*L3*sin(t2 + t3 + t4 - 1.0*t5)) - 1005.525*m6*sin(t2 + t3 + t4); (981*L3*m5*(sin(t2 + t3 + t4 - t5) + sin(t2 + t3 + t4 + t5)))/400; 0];
 end
